simulink model "Sensor_FO_TestBed"  (R2012b)
settings: Solver=ode4  StartTime=0.0  StopTime=10  RelTol=1e-3
undefined symbols (not defined in the file): MWS
libraries: Lib_Cntrl_FirstOrderSensor_TMATS x1
settings Model: Creator=jwchapm2  LastModifiedBy=jwchapm2

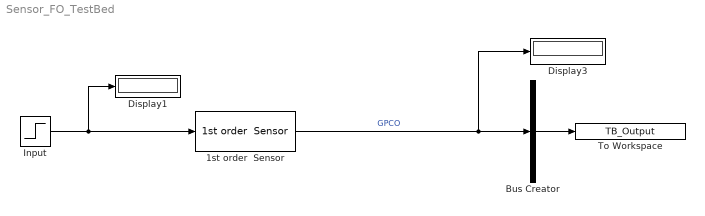
== system Sensor_FO_TestBed ==
  1st order  Sensor : Lib_Cntrl_FirstOrderSensor_TMATS/1st order  Sensor  Sen_Max_M=MWS.Sensor_FO.max  Sen_Min_M=MWS.Sensor_FO.min  Gain_M=MWS.Sensor_FO.Gain  Tau_M=MWS.Sensor_FO.Tau  GN_EN_M=on  GN_NST_M=MWS.Sensor_FO.Noise_SampleTime  F_Gain_M=MWS.Sensor_FO.FltG  F_Drift_M=MWS.Sensor_FO.FltD
  Bus Creator : BusCreator  Inputs=1
  Display1 : Display
  Display3 : Display
  Input : Step  Time=MWS.Sensor_FO.Step_Time  Before=MWS.Sensor_FO.Step_IV  After=MWS.Sensor_FO.Inp  SampleTime=0
  To Workspace : ToWorkspace  VariableName=TB_Output  SampleTime=-1
  wires:
  1st order  Sensor/1 -> Display3/1, Bus Creator/1  "GPCO"
  Bus Creator/1 -> To Workspace/1
  Input/1 -> Display1/1, 1st order  Sensor/1
